simulink model "UAM_GCS"  (R2024b)
settings: Solver=VariableStepAuto  StartTime=0.0  StopTime=10.0  RelTol=1e-3
undefined symbols (not defined in the file): CityMission, FixedWingMission, HoverMission, params, position, TransitionMission, UAVSampleTime
settings Model: DataDictionary=UAM_data.sldd  Creator=USER  LastModifiedBy=admin

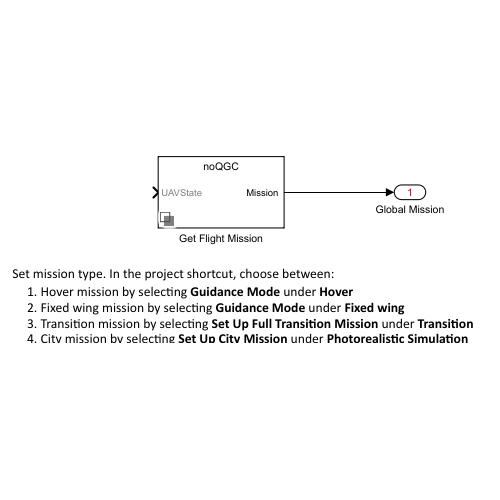
[thumbnail: Simulink's stored preview of the top-level diagram]
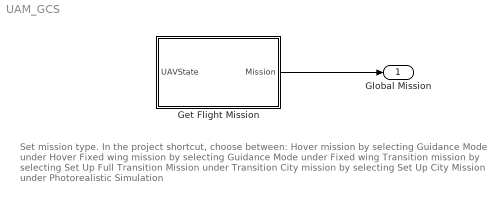
== system UAM_GCS ==
  note: Set mission type. In the project shortcut, choose between:
      | Hover mission by selecting Guidance Mode under Hover
      | Fixed wing mission by selecting Guidance Mode under Fixed wing
      | Transition mission by selecting Set Up Full Transition Mission under Transition
      | City mission by selecting Set Up City Mission under Photorealistic Simulation
  Get Flight Mission : Subsystem  Variant=on  VariantControlMode=label  LabelModeActiveChoice=useQGC==0
  Global Mission : Outport  SampleTime=0.005
  wires:
  Get Flight Mission/1("Mission ") -> Global Mission/1

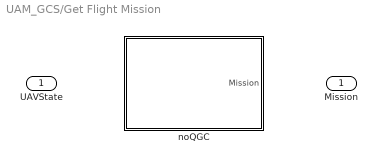
== system UAM_GCS/Get Flight Mission ==
  UAVState : Inport
  noQGC : Subsystem  TreatAsAtomicUnit=on  SystemSampleTime=UAVSampleTime*4  VariantControl=useQGC==0
  "Mission " : Outport

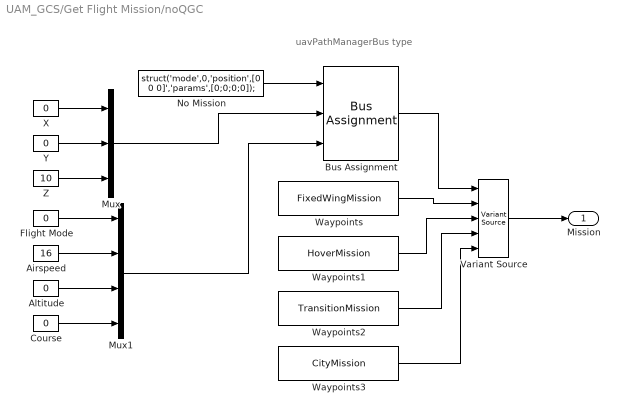
== system UAM_GCS/Get Flight Mission/noQGC ==
  note: uavPathManagerBus type
  Airspeed : Constant  Value=16
  Altitude : Constant  Value=0
  Bus Assignment : BusAssignment  AssignedSignals=position,params
  Course : Constant  Value=0
  Flight Mode : Constant  Value=0
  Mux : Mux  Inputs=3
  Mux1 : Mux
  No Mission : Constant  Value=struct('mode',0,'position',[0 0 0]','params',[0;0;0;0]);  OutDataTypeStr=Bus: doubleUavPathManager
  Variant Source : VariantSource  ShowConditionOnBlock=on
  Waypoints : Constant  Value=FixedWingMission  OutDataTypeStr=Bus: doubleUavPathManager  SampleTime=-1
  Waypoints1 : Constant  Value=HoverMission  OutDataTypeStr=Bus: doubleUavPathManager  SampleTime=-1
  Waypoints2 : Constant  Value=TransitionMission  OutDataTypeStr=Bus: doubleUavPathManager  SampleTime=-1
  Waypoints3 : Constant  Value=CityMission  OutDataTypeStr=Bus: doubleUavPathManager  SampleTime=-1
  X : Constant  Value=0
  Y : Constant  Value=0
  Z : Constant  Value=10
  Mission : Outport  PortDimensions=9
  wires:
  Waypoints/1 -> Variant Source/2
  Waypoints1/1 -> Variant Source/3
  Variant Source/1 -> Mission/1
  Waypoints2/1 -> Variant Source/4
  No Mission/1 -> Bus Assignment/1
  Waypoints3/1 -> Variant Source/5
  Bus Assignment/1 -> Variant Source/1
  X/1 -> Mux/1
  Y/1 -> Mux/2
  Z/1 -> Mux/3
  Mux/1 -> Bus Assignment/2
  Mux1/1 -> Bus Assignment/3
  Flight Mode/1 -> Mux1/1
  Course/1 -> Mux1/4
  Altitude/1 -> Mux1/3
  Airspeed/1 -> Mux1/2
